simulink model "SpacecraftDisturbances"  (Simulink 8.5)
settings: Solver=ode4  StartTime=0.0  StopTime=20000  FixedStep=1  RelTol=1e-3
InitFcn:
  | % Bifocal Relay Mirror Spacecraft (prior to payload installation) Dynamics Simulation      TA Sands
  | clear all;close all;clc;warning off all;
  | 
  | % Simulation run parameters
  | Rate=34.3; DeltaT=1/Rate;
  | 
  | % Maneuver Parameters
  | roll=0; pitch=0; yaw=30; roll=roll*pi/180; pitch=pitch*pi/180; yaw=yaw*pi/180;
  | SlewTime=5; SACengage=0;
  | 
  | %Constants0
  | Re=6371.2e3;mu=398601.2e9; %earth radius and universal gravitation constant
  | 
  | %Spacecraft orbit
  | h=300e3; %orbit altitude in meters
  | R=Re+h; %orbit radius from center of earth
  | we=0.000072921158553; %earth's angular velocity rad/solar sec(Vallado)
  | wo=sqrt(mu/(Re+h)^3); %orbit angular velocity
  | incln=36.6001*pi/180; %Inclination assumed Monterey Latitude
  | epsilon=12*pi/180; alphao=0;
  | uo=0; nuo=0; %Start S/C beneath subsolar point
  | beta=60; gamma=1.5;
  | a=0.545491852; b=0.314939867; c=0.704226952; %Assumed spacecraft rectangular size
  | Area=[b*c a*c a*b]; %projected area~m^2 in body x,y,z directions
  | density=4.39e-14;
  | kpre=-9.9639/24/3600/180*pi*0; %nodal precession constant assumed zero here
  | wn=kpre*(Re/(Re+h))^3.5*cos(incln); %nodal precession (zero eccentricity)
  | V=wo*(Re+h);
  | rho=asin(Re/(h+Re)); %earth angular radius
  | Cd=2.5; psun=4.5E-6; %Drag coefficient and solar pressure constant~N/m^2
  | Kaero=-0.5*Cd*V^2; Psolar=2*psun; %constants for aero and solar torque calculation
  | dL=[0.002 0.002 0.008]; %predicted distance between cp and cg
  | Kme=2.3390e-005;
  | 
  | %Spacecraft Magnetic Properties (assumed)
  | mresid=[0 0 0.01]; %Spacecraft residual magnetic moment
  | M=mresid; %Magnetic unit dipole vector
  | K=7.943e15;
  | MBF=K/R^3;
  | 
  | %Spacecraft Inertia conditions
  | Ix=119.1259; Iy=150.6615; Iz=106.0288;
  | Ixy=-15.76781; Iyz=22.3164; Ixz=-6.5486;
  | %Ixy=0;Iyz=0;Ixz=0;
  | Imo=[Ix Ixy Ixz;
  | Ixy Iy Iyz;
  | Ixz Iyz Iz]; %Moment of inertia matrix
  | Iinv=inv(Imo); %Moment of inertia inverse goes in dynamics block
  | 
  | %Spacecraft initial Euler state angles and rates
  | phio=0;thetao=0;psio=0; %Initial Euler Angles
  | phidoto=0;thetadoto=0;psidoto=0; %Initial Euler Rates
  | 
  | %Calculation of initial quaternion (qo) and angular momentum (Ho)
  | s1=sin(phio/2);s2=sin(thetao/2);s3=sin(psio/2);c1=cos(phio/2);c2=cos(thetao/2);c3=cos(psio/2);
  | q1o=s1*c2*c3-c1*s2*s3;
  | q2o=c1*s2*c3+s1*c2*s3; %Wie pg. 321
  | q3o=c1*c2*s3-s1*s2*c3;
  | q4o=c1*c2*c3+s1*s2*s3;
  | S1=sin(phio);S2=sin(thetao);S3=sin(psio);C1=cos(phio);C2=cos(thetao);C3=cos(psio);
  | wxo=phidoto-psidoto*S2-wo*S3*C2;
  | wyo=thetadoto*C1+psidoto*C2*S1-wo*(C3*C1+S3*S2*S1);
  | wzo=psidoto*C2*C1-thetadoto*S1-wo*(S3*S2*C1-C3*S1);
  | qo=[q1o q2o q3o q4o];
  | Ho=Imo*[wxo wyo wzo]';
  | norm(Ho)*1000;
  | 
  | %Calculate eclipse time for comparison with EPS calculations
  | Te=100.87*2*V/2/pi;
  | 
  | 
  | 
StopFcn:
  | h2=figure;
  | plot(clock,Euler),title('Not Diagonal Inertia Matrix Euler Angles'),xlabel('time(sec)'),ylabel('Angles (degrees)'),grid
  | 
  | h3=figure;
  | plot(clock,Disturbances),title('Disturbances'),xlabel('time(sec)'),ylabel('torque'),grid
  | 
  | 
  | figure(3);
  | 
  | EulerX=Euler(:,1);EulerY=Euler(:,2);EulerZ=Euler(:,3);
  | subplot(4,1,1);plot(clock,EulerX,'linewidth',3); axis([0,20000,min(EulerX)-0.01,max(EulerX)+0.01]);grid;ylabel('\phi(deg)','fontsize',14);title('True Euler Angles','fontsize',14); set(gca,'XTickLabel',{' ',' ',' ',' ',' ',' ',' ',' ','15'}); set(gca,'fontsize',16);
  | subplot(4,1,2);plot(clock,EulerY,'linewidth',3); axis([0,20000,min(EulerY)-0.01,max(EulerY)+0.01]); grid;ylabel('\theta(deg)','fontsize',14); set(gca,'XTickLabel',{' ',' ',' ',' ',' ',' ',' ',' ','15'}); set(gca,'fontsize',16);
  | subplot(4,1,3);plot(clock,EulerZ,'linewidth',3);axis([0,20000,min(EulerZ)-0.01,max(EulerZ)+0.01]);grid; ylabel('\psi(deg)','fontsize',14); set(gca,'XTickLabel',{' ',' ',' ',' ',' ',' ',' ',' ','15'}); set(gca,'fontsize',16);
  | 
  | EX=ERROR(:,1); EY=ERROR(:,2); EZ=ERROR(:,3);
  | MeanXerror=mean(EX); Xmean=num2str(MeanXerror); xmean=['\mu_\phi=', Xmean];
  | STDx=std(EX);Xsigma=num2str(STDx);SigmaX=[' \sigma_x=' Xsigma]; xlegend=[xmean, SigmaX];
  | MeanYerror=mean(EY); Ymean=num2str(MeanYerror); ymean=['\mu_\theta=', Ymean];
  | STDy=std(EY); Ysigma=num2str(STDy);SigmaY=[' \sigma_y=' Ysigma]; ylegend=[ymean, SigmaY];
  | MeanZerror=mean(EZ); Zmean=num2str(MeanZerror); zmean=['\mu_\psi=', Zmean];
  | STDz=std(EZ);Zsigma=num2str(STDz);SigmaZ=[' \sigma_z=' Zsigma]; zlegend=[zmean, SigmaZ];
  | MeanError=[MeanXerror MeanYerror MeanZerror]; StdDev=[STDx STDy STDz];
  | 
  | 
  | subplot(4,1,1);plot(clock,EulerX,'linewidth',2); axis([0,20000,min(EulerX)-0.01,max(EulerX)+0.01]);grid;ylabel('\phi(deg)','fontsize',10);title('Standard Deviation Euler Angles','fontsize',14); set(gca,'XTickLabel',{' ',' ',' ',' ',' ',' ',' ',' ','10'}); set(gca,'fontsize',10);
  | subplot(4,1,2);plot(clock,EulerY,'linewidth',2); axis([0,20000,min(EulerY)-0.01,max(EulerY)+0.01]); grid;ylabel('\theta(deg)','fontsize',10); set(gca,'XTickLabel',{' ',' ',' ',' ',' ',' ',' ',' ','10'}); set(gca,'fontsize',10);
  | subplot(4,1,3);plot(clock,EulerZ,'linewidth',2);axis([0,20000,min(EulerZ)-0.01,max(EulerZ)+0.01]);grid; ylabel('\psi(deg)','fontsize',10); set(gca,'XTickLabel',{' ',' ',' ',' ',' ',' ',' ',' ','10'}); set(gca,'fontsize',10);
  | subplot(4,1,4);plot(clock,EulerX,'linewidth',2);axis([0,20000,min(EulerZ)-0.01,max(EulerZ)+0.01]);grid; ylabel('\psi(deg)','fontsize',10); set(gca,'XTickLabel',{' ',' ',' ',' ',' ',' ',' ',' ','10'}); set(gca,'fontsize',10);
  | 
  | 
  | figure(7);
  | 
  | EulerX=Euler(:,1);EulerY=Euler(:,2);EulerZ=Euler(:,3);
  | 
  | subplot(3,1,1);plot(clock,EulerX,'linewidth',1.5); axis([0,20000,min(EulerX)-10,max(EulerX)+10]);grid;ylabel('roll(deg)','fontsize',10);title('Euler Angles','fontsize',14); set(gca,'XTickLabel'); set(gca,'fontsize',10);
  | subplot(3,1,2);plot(clock,EulerY,'linewidth',1.5); axis([0,20000,min(EulerY)-10,max(EulerY)+10]); grid;ylabel('pitch(deg)','fontsize',10); set(gca,'XTickLabel'); set(gca,'fontsize',10);
  | subplot(3,1,3);plot(clock,EulerZ,'linewidth',1.5);axis([0,20000,min(EulerZ)-10,max(EulerZ)+10]);grid; ylabel('yaw(deg)','fontsize',10); set(gca,'XTickLabel'); set(gca,'fontsize',10);
  | 
  | figure(8);
  | 
  | DistX=Disturbances(:,1);DistY=Disturbances(:,2);DistZ=Disturbances(:,3);
  | 
  | subplot(3,1,1);plot(clock,DistX,'linewidth',1.5); axis([0,20000,min(DistX)-0.000001,max(DistX)+0.000001]);grid;ylabel('roll(deg)','fontsize',10);title('Disturbances','fontsize',14); set(gca,'XTickLabel'); set(gca,'fontsize',10);
  | subplot(3,1,2);plot(clock,DistY,'linewidth',1.5);axis([0,20000,min(DistY)-0.000001,max(DistY)+0.000001]);grid; ylabel('pitch(deg)','fontsize',10); set(gca,'XTickLabel'); set(gca,'fontsize',10);
  | subplot(3,1,3);plot(clock,DistZ,'linewidth',1.5);axis([0,20000,min(DistZ)-0.000001,max(DistZ)+0.000001]);grid; ylabel('yaw(deg)','fontsize',10); set(gca,'XTickLabel'); set(gca,'fontsize',10);
  | 
  | figure(9);
  | 
  | GravX=Gravity(:,1);GravY=Gravity(:,2);GravZ=Gravity(:,3);
  | 
  | subplot(3,1,1);plot(clock,GravX,'linewidth',1.5); axis([0,20000,min(GravX)-0.000001,max(GravX)+0.000001]);grid;ylabel('roll(deg)','fontsize',10);title('Gravity Gradient','fontsize',14); set(gca,'XTickLabel'); set(gca,'fontsize',10);
  | subplot(3,1,2);plot(clock,GravY,'linewidth',1.5);axis([0,20000,min(GravY)-0.000001,max(GravY)+0.000001]);grid; ylabel('pitch(deg)','fontsize',10); set(gca,'XTickLabel'); set(gca,'fontsize',10);
  | subplot(3,1,3);plot(clock,GravZ,'linewidth',1.5);axis([0,20000,min(GravZ)-0.000001,max(GravZ)+0.000001]);grid; ylabel('yaw(deg)','fontsize',10); set(gca,'XTickLabel'); set(gca,'fontsize',10);
  | 
  | figure(10);
  | 
  | MagX=Magnetic(:,1);MagY=Magnetic(:,2);MagZ=Magnetic(:,3);
  | 
  | subplot(3,1,1);plot(clock,MagX,'linewidth',1.5); axis([0,20000,min(MagX)-0.000000001,max(MagX)+0.000000001]);grid;ylabel('roll(deg)','fontsize',10);title('Magnetic Torque','fontsize',14); set(gca,'XTickLabel'); set(gca,'fontsize',10);
  | subplot(3,1,2);plot(clock,MagY,'linewidth',1.5);axis([0,20000,min(MagY)-0.000000001,max(MagY)+0.000000001]);grid; ylabel('pitch(deg)','fontsize',10); set(gca,'XTickLabel'); set(gca,'fontsize',10);
  | subplot(3,1,3);plot(clock,MagZ,'linewidth',1.5);axis([0,20000,min(MagZ)-0.000000001,max(MagZ)+0.000000001]);grid; ylabel('yaw(deg)','fontsize',10); set(gca,'XTickLabel'); set(gca,'fontsize',10);
  | 
  | figure(11);
  | 
  | ASX=AeroSolar(:,1);ASY=AeroSolar(:,2);ASZ=AeroSolar(:,3);
  | 
  | subplot(3,1,1);plot(clock,ASX,'linewidth',1.5); axis([0,20000,min(ASX)-0.000001,max(ASX)+0.000001]);grid;ylabel('roll(deg)','fontsize',10);title('AeroDynamic & Solar Disturbances','fontsize',14); set(gca,'XTickLabel'); set(gca,'fontsize',10);
  | subplot(3,1,2);plot(clock,ASY,'linewidth',1.5);axis([0,20000,min(ASY)-0.000001,max(ASY)+0.000001]);grid; ylabel('pitch(deg)','fontsize',10); set(gca,'XTickLabel'); set(gca,'fontsize',10);
  | subplot(3,1,3);plot(clock,ASZ,'linewidth',1.5);axis([0,20000,min(ASZ)-0.000001,max(ASZ)+0.000001]);grid; ylabel('yaw(deg)','fontsize',10); set(gca,'XTickLabel'); set(gca,'fontsize',10);
  | 
  | figure(11);
  | 
  | AX=Gravity(:,1);AY=Magnetic(:,1);AZ=AeroSolar(:,1);
  | 
  | subplot(3,1,1);plot(clock,AX,'linewidth',1.5); axis([0,20000,min(AX),max(AX)]);grid;ylabel('Gravity','fontsize',10);title('Disturbances on Roll','fontsize',14); set(gca,'XTickLabel'); set(gca,'fontsize',10);
  | subplot(3,1,2);plot(clock,AY,'linewidth',1.5);axis([0,20000,min(AY),max(AY)]);grid; ylabel('Magnetic','fontsize',10); set(gca,'XTickLabel'); set(gca,'fontsize',10);
  | subplot(3,1,3);plot(clock,AZ,'linewidth',1.5);axis([0,20000,min(AZ),max(AZ)]);grid; ylabel('Aerosolar','fontsize',10); set(gca,'XTickLabel'); set(gca,'fontsize',10);
  | 
  | figure(5);
  | 
  | DX=art(:,2);DY=art(:,3);DZ=art(:,4);
  | 
  | subplot(3,1,1);plot(clock,DX,'linewidth',1.5); axis([0,20000,min(DX)-0.000001,max(DX)+0.000001]);grid;ylabel('step','fontsize',10);title('Disturbances','fontsize',14); set(gca,'XTickLabel'); set(gca,'fontsize',10);
  | subplot(3,1,2);plot(clock,DY,'linewidth',1.5);axis([0,20000,min(DY)-0.000001,max(DY)+0.000001]);grid; ylabel('pulse','fontsize',10); set(gca,'XTickLabel'); set(gca,'fontsize',10);
  | subplot(3,1,3);plot(clock,DZ,'linewidth',1.5);axis([0,20000,min(DZ)-0.000001,max(DZ)+0.000001]);grid; ylabel('sine','fontsize',10); set(gca,'XTickLabel'); set(gca,'fontsize',10);
  | 
  | 
  | figure(14)
  | 
  | subplot(3,1,1) ;plot(clock,ERROR(:,1)*180/pi,'linewidth',3); set(gca,'fontsize',10);title('Euler Angles','fontsize',14); ylabel('\phi Degrees','fontsize',10);
  | legend(['angle','  \mu=',num2str(mean(ERROR(:,1))),'  \sigma=',num2str(std(ERROR(:,1)))],'Location','Best')
  | legend('boxoff')
  | grid on
  | set(gca,'XTickLabel',{})
  | 
  | subplot(3,1,2) ;plot(clock,ERROR(:,2)*180/pi,'linewidth',3) ;set(gca,'fontsize',10);ylabel('\theta Degrees','fontsize',10) ;
  | legend(['angle','  \mu=',num2str(mean(ERROR(:,2))),'  \sigma=',num2str(std(ERROR(:,2)))],'Location','Best') ;
  | legend('boxoff')
  | grid on
  | set(gca,'XTickLabel',{})
  | 
  | subplot(3,1,3) ;plot(clock,ERROR(:,3)*180/pi,'linewidth',3) ;set(gca,'fontsize',10);ylabel('\psi Degrees','fontsize',10) ;xlabel('Time (s)','fontsize',10) ;
  | legend(['angle','  \mu=',num2str(mean(ERROR(:,3))),'  \sigma=',num2str(std(ERROR(:,3)))],'Location','Best')
  | legend('boxoff')
  | grid on
libraries: aerospace x4, vrlib x1, simulink x1
settings Model: Creator=grompone  LastModifiedBy=Acer
settings OptimizationCC: InitFltsAndDblsToZero=on
settings DebuggingCC: SaveWithParameterizedLinksMsg=none  SolverPrmCheckMsg=warning  FcnCallInpInsideContextMsg=UseLocalSettings  StrictBusMsg=Warning
settings SFSimCC: SimParseCustomCode=off
settings GRTTargetCC: TargetFcnLib=ansi_tfl_tmw.mat

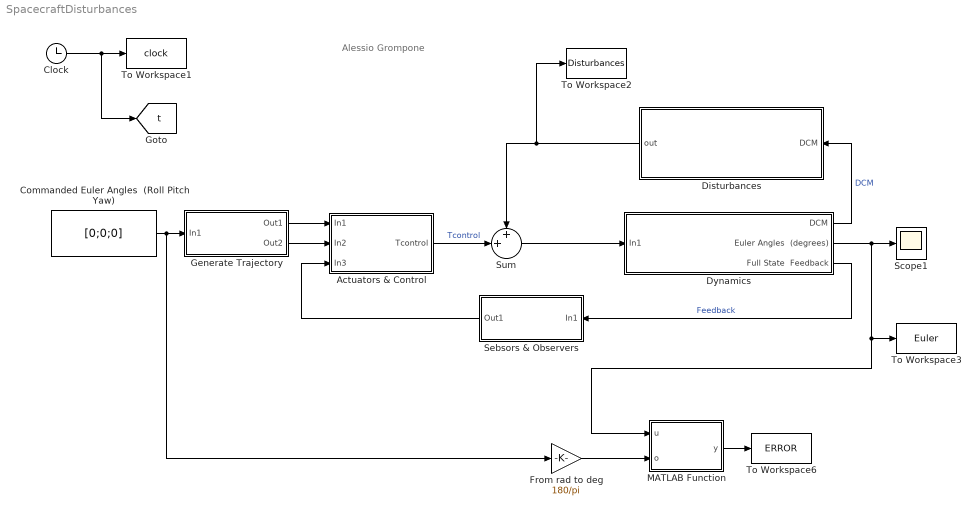
== system SpacecraftDisturbances ==
  note: Alessio Grompone
  Actuators & Control : Subsystem
  Clock : Clock
  Commanded Euler Angles  (Roll Pitch Yaw) : Constant  Value=[0;0;0]
  Disturbances : Subsystem
  Dynamics : Subsystem
  From rad to deg : Gain  Gain=180/pi
  Generate Trajectory : Subsystem
  MATLAB Function : MATLAB Function  TreatAsAtomicUnit=on
  Scope1 : Scope
      settings: SaveName=ScopeData2
  Sebsors & Observers : Subsystem
  Sum : Sum  Inputs=++|
  To Workspace1 : ToWorkspace  VariableName=clock  SampleTime=-1
  To Workspace2 : ToWorkspace  VariableName=Disturbances  SampleTime=-1
  To Workspace3 : ToWorkspace  VariableName=Euler  SampleTime=-1
  To Workspace6 : ToWorkspace  VariableName=ERROR  SampleTime=-1
  tag scope: t=global
  wires:
  Clock/1 -> To Workspace1/1, [t]
  Sum/1 -> Dynamics/1(In1)
  Commanded Euler Angles  (Roll Pitch Yaw)/1 -> Generate Trajectory/1(In1), From rad to deg/1
  Generate Trajectory/1(Out1) -> Actuators & Control/1(In1)
  Generate Trajectory/2(Out2) -> Actuators & Control/2(In2)
  Sebsors & Observers/1(Out1) -> Actuators & Control/3(In3)
  Dynamics/2(Euler Angles  (degrees)) -> Scope1/1, To Workspace3/1, MATLAB Function/1(u)
  Dynamics/1(DCM) -> Disturbances/1(DCM)  "DCM"
  Dynamics/3(Full State  Feedback) -> Sebsors & Observers/1(In1)  "Feedback"
  Disturbances/1(out) -> Sum/1, To Workspace2/1
  Actuators & Control/1(Tcontrol) -> Sum/2  "Tcontrol"
  MATLAB Function/1(y) -> To Workspace6/1
  From rad to deg/1 -> MATLAB Function/2(o)

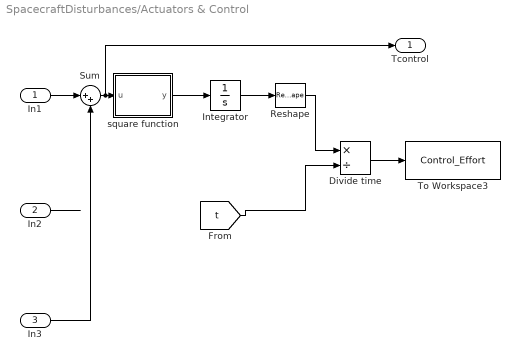
== system SpacecraftDisturbances/Actuators & Control ==
  In1 : Inport
  In2 : Inport  Port=2
  In3 : Inport  Port=3
  Divide time : Product  Inputs=*/
  Integrator : Integrator
  Reshape : Reshape
  Sum : Sum  Inputs=|++
  To Workspace3 : ToWorkspace  VariableName=Control_Effort  SampleTime=-1
  square function : MATLAB Function  TreatAsAtomicUnit=on
  Tcontrol : Outport
  wires:
  [t] -> Divide time/2
  square function/1(y) -> Integrator/1
  Integrator/1 -> Reshape/1
  Divide time/1 -> To Workspace3/1
  Reshape/1 -> Divide time/1
  In2/1 -> ?
  In1/1 -> Sum/1
  In3/1 -> Sum/2
  Sum/1 -> square function/1(u), Tcontrol/1

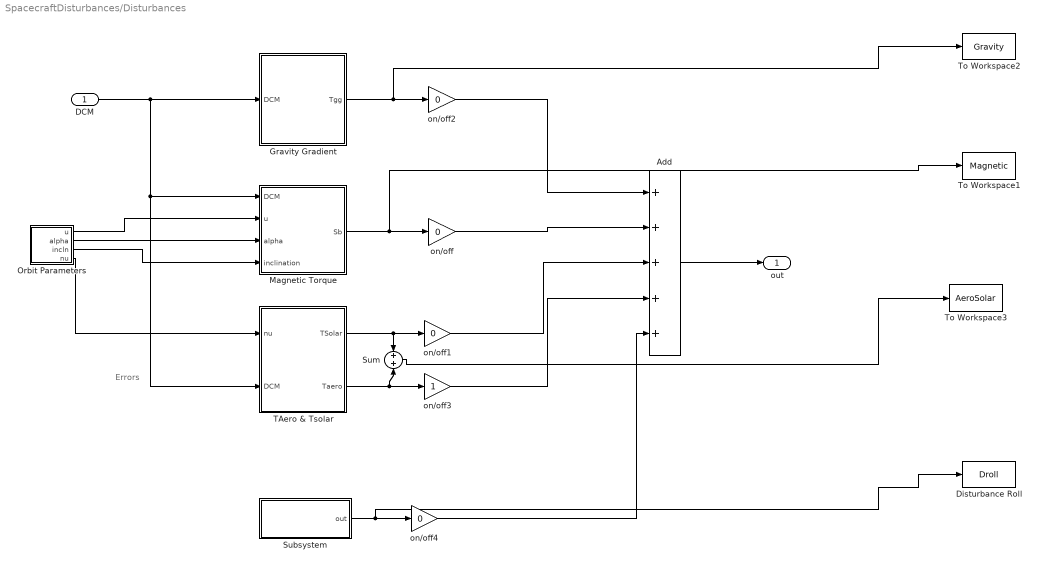
== system SpacecraftDisturbances/Disturbances ==
  note: Errors
  DCM : Inport
  Add : Sum  Inputs=+++++
  Disturbance Roll : ToWorkspace  VariableName=Droll  SampleTime=-1
  Gravity Gradient : Subsystem
  Magnetic Torque : Subsystem
  Orbit Parameters : Subsystem
  Subsystem : Subsystem
  Sum : Sum  Inputs=+|+
  TAero & Tsolar : Subsystem
  To Workspace1 : ToWorkspace  VariableName=Magnetic  SampleTime=-1
  To Workspace2 : ToWorkspace  VariableName=Gravity  SampleTime=-1
  To Workspace3 : ToWorkspace  VariableName=AeroSolar  SampleTime=-1
  on/off{,1..2,4} (4 alike) : Gain  Gain=0
  on/off3 : Gain
  out : Outport
  wires:
  DCM/1 -> Magnetic Torque/1(DCM), TAero & Tsolar/2(DCM), Gravity Gradient/1(DCM)
  TAero & Tsolar/1(TSolar) -> on/off1/1, Sum/1
  Magnetic Torque/1(Sb) -> on/off/1, To Workspace1/1
  Orbit Parameters/1(u) -> Magnetic Torque/2(u)
  Orbit Parameters/2(alpha) -> Magnetic Torque/3(alpha)
  Orbit Parameters/3(incln) -> Magnetic Torque/4(inclination)
  Orbit Parameters/4(nu) -> TAero & Tsolar/1(nu)
  Gravity Gradient/1(Tgg) -> on/off2/1, To Workspace2/1
  Add/1 -> out/1
  on/off2/1 -> Add/1
  on/off/1 -> Add/2
  TAero & Tsolar/2(Taero) -> on/off3/1, Sum/2
  on/off1/1 -> Add/3
  on/off3/1 -> Add/4
  Subsystem/1(out) -> on/off4/1, Disturbance Roll/1
  on/off4/1 -> Add/5
  Sum/1 -> To Workspace3/1

== system SpacecraftDisturbances/Dynamics ==
  In1 : Inport
  Dynamics : Subsystem
  Kinematics : Subsystem
  Mux : Mux  Inputs=2
  DCM : Outport
  Euler Angles  (degrees) : Outport  Port=2
  Full State  Feedback : Outport  Port=3
  wires:
  Dynamics/1(w_nb) -> Kinematics/1(w_nb), Mux/2
  Kinematics/1(DCM) -> DCM/1
  In1/1 -> Dynamics/1(taug)
  Kinematics/2(Euler Angles  (degrees)) -> Euler Angles  (degrees)/1
  Mux/1 -> Full State  Feedback/1
  Kinematics/3(Euler Angles) -> Mux/1

== system SpacecraftDisturbances/Generate Trajectory ==
  In1 : Inport
  Out1 : Outport
  Out2 : Outport  Port=2
  wires:
  In1/1 -> Out1/1

== system SpacecraftDisturbances/Sebsors & Observers ==
  In1 : Inport
  Demux : Demux  Outputs=6
  Mux : Mux  Inputs=3
  Out1 : Outport
  wires:
  Mux/1 -> Out1/1
  Demux/1 -> Mux/1
  Demux/2 -> Mux/2
  Demux/3 -> Mux/3

== system SpacecraftDisturbances/Disturbances/Gravity Gradient ==
  DCM : Inport
  3*mu/Ro^3 : Gain  Gain=3*mu/(h+Re)^3  Multiplication=Matrix(K*u)  SaturateOnIntegerOverflow=on  OutDataTypeStr=Inherit: Same as input  ParamDataTypeStr=Inherit: Same as input
  3x3 cross product : aerospace/Axes Transformations/3x3 cross product
  Ib : Gain  Gain=Imo  Multiplication=Matrix(K*u)  SaturateOnIntegerOverflow=on  OutDataTypeStr=Inherit: Same as input  ParamDataTypeStr=Inherit: Same as input
  Select ci3 : Subsystem
  Tgg : Outport
  wires:
  Ib/1 -> 3x3 cross product/2
  3*mu/Ro^3/1 -> Tgg/1
  3x3 cross product/1 -> 3*mu/Ro^3/1
  Select ci3/1(U(E)) -> 3x3 cross product/1, Ib/1
  DCM/1 -> Select ci3/1(U)

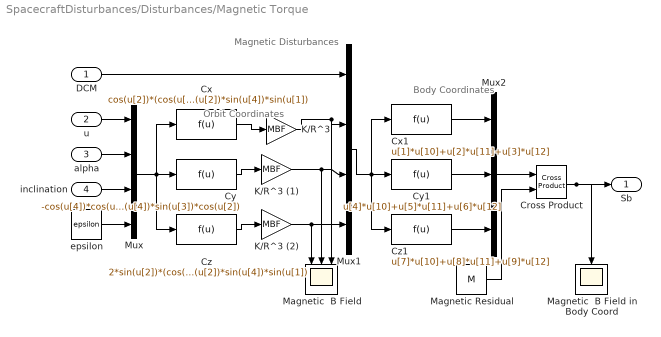
== system SpacecraftDisturbances/Disturbances/Magnetic Torque ==
  note: Magnetic Disturbances
  note: Orbit Coordinates
  note: Body Coordinates
  DCM : Inport
  u : Inport  Port=2
  alpha : Inport  Port=3
  inclination : Inport  Port=4
  Cross Product : vrlib/Utilities/Cross Product
  Cx : Fcn  Expr=cos(u[2])*(cos(u[4])*sin(u[3])-sin(u[4])*cos(u[3])*cos(u[1]))-sin(u[2])*sin(u[4])*sin(u[1])
  Cx1 : Fcn  Expr=u[1]*u[10]+u[2]*u[11]+u[3]*u[12]
  Cy : Fcn  Expr=-cos(u[4])*cos(u[3])-sin(u[4])*sin(u[3])*cos(u[2])
  Cy1 : Fcn  Expr=u[4]*u[10]+u[5]*u[11]+u[6]*u[12]
  Cz : Fcn  Expr=2*sin(u[2])*(cos(u[4])*sin(u[3])-sin(u[4])*cos(u[3])*cos(u[1]))+2*cos(u[2])*sin(u[4])*sin(u[1])
  Cz1 : Fcn  Expr=u[7]*u[10]+u[8]*u[11]+u[9]*u[12]
  K/R^3 : Gain  Gain=MBF
  K/R^3 (1) : Gain  Gain=MBF
  K/R^3 (2) : Gain  Gain=MBF
  Magnetic Residual : Constant  Value=M
  Magnetic  B Field : Scope  NumInputPorts=3
      settings: YMin=-5~-5~-5  YMax=5~5~5  SaveName=ScopeData3
  Magnetic  B Field in Body Coord : Scope
      settings: SaveName=ScopeData4
  Mux : Mux
  Mux1 : Mux
  Mux2 : Mux  Inputs=3
  epsilon : Constant  Value=epsilon
  Sb : Outport
  wires:
  u/1 -> Mux/1
  inclination/1 -> Mux/3
  alpha/1 -> Mux/2
  Cx/1 -> K/R^3/1
  Cy/1 -> K/R^3 (1)/1
  Cz/1 -> K/R^3 (2)/1
  DCM/1 -> Mux1/1
  Mux/1 -> Cy/1, Cz/1, Cx/1
  K/R^3/1 -> Mux1/2, Magnetic  B Field/3
  K/R^3 (1)/1 -> Mux1/3, Magnetic  B Field/2
  K/R^3 (2)/1 -> Mux1/4, Magnetic  B Field/1
  epsilon/1 -> Mux/4
  Mux1/1 -> Cy1/1, Cz1/1, Cx1/1
  Cx1/1 -> Mux2/1
  Cy1/1 -> Mux2/2
  Cz1/1 -> Mux2/3
  Magnetic Residual/1 -> Cross Product/2
  Mux2/1 -> Cross Product/1
  Cross Product/1 -> Sb/1, Magnetic  B Field in Body Coord/1

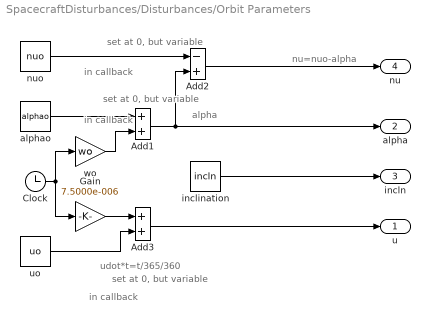
== system SpacecraftDisturbances/Disturbances/Orbit Parameters ==
  note: nu=nuo-alpha
  note: alpha
  note: udot*t=t/365/360
  note: set at 0, but variable
  note: in callback
  note: set at 0, but variable
  note: in callback
  note: set at 0, but variable
  note: in callback
  Add1 : Sum
  Add2 : Sum  Inputs=-+
  Add3 : Sum
  Clock : Clock
  Gain : Gain  Gain=7.5000e-006
  alphao : Constant  Value=alphao
  inclination : Constant  Value=incln
  nuo : Constant  Value=nuo
  uo : Constant  Value=uo
  wo : Gain  Gain=wo
  u : Outport
  alpha : Outport  Port=2
  incln : Outport  Port=3
  nu : Outport  Port=4
  wires:
  nuo/1 -> Add2/1
  Add2/1 -> nu/1
  alphao/1 -> Add1/1
  Clock/1 -> wo/1, Gain/1
  wo/1 -> Add1/2
  Add1/1 -> alpha/1, Add2/2
  uo/1 -> Add3/2
  Gain/1 -> Add3/1
  inclination/1 -> incln/1
  Add3/1 -> u/1

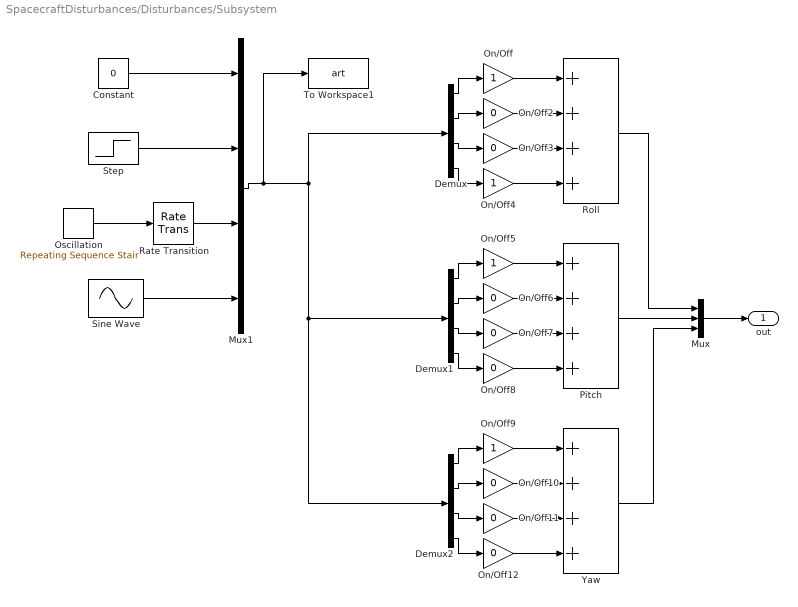
== system SpacecraftDisturbances/Disturbances/Subsystem ==
  Constant : Constant  Value=0
  Demux : Demux
  Demux1 : Demux
  Demux2 : Demux
  Mux : Mux  Inputs=3
  Mux1 : Mux
  On/Off{,4..5,9} (4 alike) : Gain  SaturateOnIntegerOverflow=on  OutDataTypeStr=Inherit: Same as input  ParamDataTypeStr=Inherit: Same as input
  On/Off{2..3,6..8,10..12} (8 alike) : Gain  Gain=0  SaturateOnIntegerOverflow=on  OutDataTypeStr=Inherit: Same as input  ParamDataTypeStr=Inherit: Same as input
  Oscillation : simulink/Sources/Repeating Sequence Stair  OutValues=[ 0.01 -0.01 -0.01 0.01]  tsamp=1000  OutMin=[]  OutMax=[]  OutDataTypeStr=double  OutputDataTypeScalingMode=double  OutDataType=fixdt(0,8)  ConRadixGroup=Best Precision: Vector-wise  OutScaling=2^-12
  Pitch : Sum  Inputs=++++
  Rate Transition : RateTransition
  Roll : Sum  Inputs=++++
  Sine Wave : Sin  Amplitude=.1  Frequency=1000  SampleTime=0  VectorParams1D=off
  Step : Step  Time=4000  After=0.1  SampleTime=0
  To Workspace1 : ToWorkspace  VariableName=art  SampleTime=-1
  Yaw : Sum  Inputs=++++
  out : Outport
  wires:
  On/Off/1 -> Roll/1
  On/Off2/1 -> Roll/2
  On/Off3/1 -> Roll/3
  On/Off4/1 -> Roll/4
  On/Off5/1 -> Pitch/1
  On/Off6/1 -> Pitch/2
  On/Off7/1 -> Pitch/3
  On/Off8/1 -> Pitch/4
  On/Off9/1 -> Yaw/1
  On/Off10/1 -> Yaw/2
  On/Off11/1 -> Yaw/3
  On/Off12/1 -> Yaw/4
  Roll/1 -> Mux/1
  Pitch/1 -> Mux/2
  Yaw/1 -> Mux/3
  Demux/1 -> On/Off/1
  Demux/2 -> On/Off2/1
  Demux/3 -> On/Off3/1
  Demux/4 -> On/Off4/1
  Demux1/1 -> On/Off5/1
  Demux1/2 -> On/Off6/1
  Demux1/3 -> On/Off7/1
  Demux1/4 -> On/Off8/1
  Demux2/1 -> On/Off9/1
  Demux2/2 -> On/Off10/1
  Demux2/3 -> On/Off11/1
  Demux2/4 -> On/Off12/1
  Constant/1 -> Mux1/1
  Step/1 -> Mux1/2
  Mux/1 -> out/1
  Mux1/1 -> Demux/1, Demux1/1, Demux2/1, To Workspace1/1
  Sine Wave/1 -> Mux1/4
  Rate Transition/1 -> Mux1/3
  Oscillation/1 -> Rate Transition/1

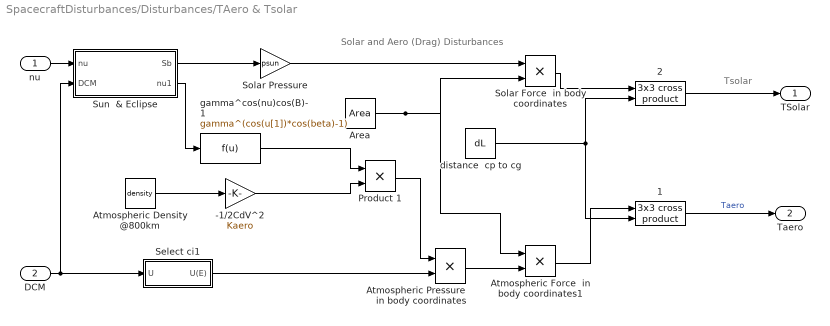
== system SpacecraftDisturbances/Disturbances/TAero & Tsolar ==
  note: Tsolar
  note: Solar and Aero (Drag) Disturbances
  nu : Inport
  DCM : Inport  Port=2
  -1/2CdV^2 : Gain  Gain=Kaero
  1 : aerospace/Axes Transformations/3x3 cross product
  2 : aerospace/Axes Transformations/3x3 cross product
  Area : Constant  Value=Area
  Atmospheric Density @800km : Constant  Value=density
  Atmospheric Force  in body coordinates1 : Product  RndMeth=Zero
  Atmospheric Pressure in body coordinates : Product  RndMeth=Zero
  Product 1 : Product  RndMeth=Zero
  Select ci1 : Subsystem
  Solar Force  in body coordinates : Product  RndMeth=Zero
  Solar Pressure : Gain  Gain=psun
  Sun  & Eclipse : Subsystem
  distance  cp to cg : Constant  Value=dL
  gamma^cos(nu)cos(B)-1 : Fcn  Expr=gamma^(cos(u[1])*cos(beta)-1)
  TSolar : Outport
  Taero : Outport  Port=2
  wires:
  DCM/1 -> Select ci1/1(U), Sun  & Eclipse/2(DCM)
  nu/1 -> Sun  & Eclipse/1(nu)
  Sun  & Eclipse/1(Sb) -> Solar Pressure/1
  Sun  & Eclipse/2(nu1) -> gamma^cos(nu)cos(B)-1/1
  Solar Pressure/1 -> Solar Force  in body coordinates/1
  gamma^cos(nu)cos(B)-1/1 -> Product 1/1
  Atmospheric Pressure in body coordinates/1 -> Atmospheric Force  in body coordinates1/2
  Atmospheric Density @800km/1 -> -1/2CdV^2/1
  -1/2CdV^2/1 -> Product 1/2
  Area/1 -> Solar Force  in body coordinates/2, Atmospheric Force  in body coordinates1/1
  Select ci1/1(U(E)) -> Atmospheric Pressure in body coordinates/2
  Product 1/1 -> Atmospheric Pressure in body coordinates/1
  Solar Force  in body coordinates/1 -> 2/1
  distance  cp to cg/1 -> 2/2, 1/2
  2/1 -> TSolar/1
  1/1 -> Taero/1  "Taero"
  Atmospheric Force  in body coordinates1/1 -> 1/1

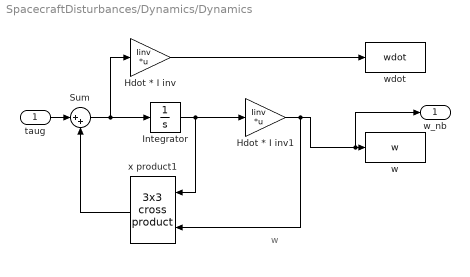
== system SpacecraftDisturbances/Dynamics/Dynamics ==
  note: w
  taug : Inport
  "  Hdot * I inv" : Gain  Gain=Iinv  Multiplication=Matrix(K*u)  SaturateOnIntegerOverflow=on  OutDataTypeStr=Inherit: Same as input  ParamDataTypeStr=Inherit: Same as input
  "  Hdot * I inv1" : Gain  Gain=Iinv  Multiplication=Matrix(K*u)  SaturateOnIntegerOverflow=on  OutDataTypeStr=Inherit: Same as input  ParamDataTypeStr=Inherit: Same as input
  Integrator : Integrator
  Sum : Sum  Inputs=|++
  w : ToWorkspace  VariableName=w  SampleTime=-1
  wdot : ToWorkspace  VariableName=wdot  SampleTime=-1
  x product1 : aerospace/Axes Transformations/3x3 cross product
  w_nb : Outport
  wires:
  Integrator/1 -> x product1/1, "  Hdot * I inv1"/1
  taug/1 -> Sum/1
  x product1/1 -> Sum/2
  Sum/1 -> "  Hdot * I inv"/1, Integrator/1
  "  Hdot * I inv"/1 -> wdot/1
  "  Hdot * I inv1"/1 -> x product1/2, w/1, w_nb/1

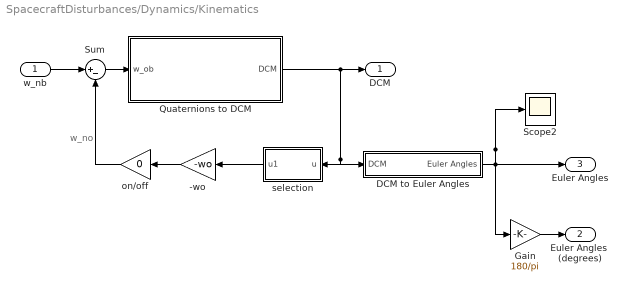
== system SpacecraftDisturbances/Dynamics/Kinematics ==
  note: w_no
  w_nb : Inport
  -wo : Gain  Gain=-wo
  DCM to Euler Angles : Subsystem
  Gain : Gain  Gain=180/pi
  Quaternions to DCM : Subsystem
  Scope2 : Scope
      settings: YMin=-60  YMax=60  SaveName=ScopeData3
  Sum : Sum  Inputs=|+-
  on/off : Gain  Gain=0
  "selection " : MATLAB Function  TreatAsAtomicUnit=on
  DCM : Outport
  Euler Angles  (degrees) : Outport  Port=2
  Euler Angles : Outport  Port=3
  wires:
  w_nb/1 -> Sum/1
  Quaternions to DCM/1(DCM) -> DCM/1, "selection "/1(u), DCM to Euler Angles/1(DCM)
  Sum/1 -> Quaternions to DCM/1(w_ob)
  on/off/1 -> Sum/2
  "selection "/1(u1) -> -wo/1
  -wo/1 -> on/off/1
  Gain/1 -> Euler Angles  (degrees)/1
  DCM to Euler Angles/1(Euler Angles) -> Scope2/1, Euler Angles/1, Gain/1

== system SpacecraftDisturbances/Disturbances/Gravity Gradient/Select ci3 ==
  U : Inport
  C13 : Fcn  Expr=u[3]
  C23 : Fcn  Expr=u[6]
  C33 : Fcn  Expr=u[9]
  Mux2 : Mux  Inputs=3
  U(E) : Outport
  wires:
  Mux2/1 -> U(E)/1
  U/1 -> C33/1, C13/1, C23/1
  C33/1 -> Mux2/3
  C23/1 -> Mux2/2
  C13/1 -> Mux2/1

== system SpacecraftDisturbances/Disturbances/TAero & Tsolar/Select ci1 ==
  U : Inport
  C13 : Fcn  Expr=u[1]
  C23 : Fcn  Expr=u[4]
  C33 : Fcn  Expr=u[7]
  Mux : Mux  Inputs=3
  U(E) : Outport
  wires:
  C23/1 -> Mux/2
  C13/1 -> Mux/1
  C33/1 -> Mux/3
  Mux/1 -> U(E)/1
  U/1 -> C13/1, C23/1, C33/1

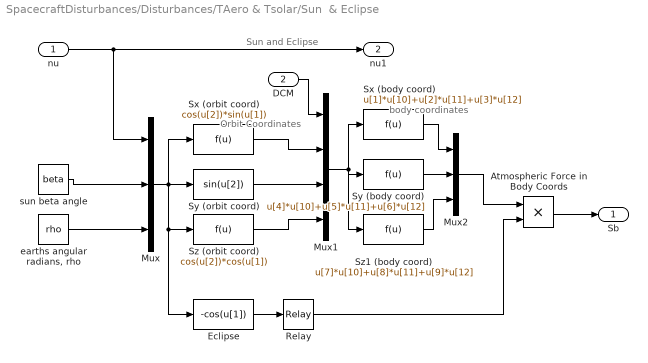
== system SpacecraftDisturbances/Disturbances/TAero & Tsolar/Sun  & Eclipse ==
  note: Sun and Eclipse
  note: Orbit Coordinates
  note: body coordinates
  nu : Inport
  DCM : Inport  Port=2
  Atmospheric Force in Body Coords : Product  RndMeth=Zero
  Eclipse : Fcn  Expr=-cos(u[1])
  Mux : Mux  Inputs=3
  Mux1 : Mux
  Mux2 : Mux  Inputs=3
  Relay : Relay  OnSwitchValue=cos(rho)/cos(beta)  OffSwitchValue=cos(rho)/cos(beta)-0.001  OnOutputValue=0  OffOutputValue=1
  Sx (body coord) : Fcn  Expr=u[1]*u[10]+u[2]*u[11]+u[3]*u[12]
  Sx (orbit coord) : Fcn  Expr=cos(u[2])*sin(u[1])
  Sy (body coord) : Fcn  Expr=u[4]*u[10]+u[5]*u[11]+u[6]*u[12]
  "Sy (orbit coord) " : Fcn  Expr=sin(u[2])
  Sz (orbit coord) : Fcn  Expr=cos(u[2])*cos(u[1])
  Sz1 (body coord) : Fcn  Expr=u[7]*u[10]+u[8]*u[11]+u[9]*u[12]
  "earths angular radians, rho" : Constant  Value=rho
  sun beta angle : Constant  Value=beta
  Sb : Outport
  nu1 : Outport  Port=2
  wires:
  Mux1/1 -> Sx (body coord)/1, Sy (body coord)/1, Sz1 (body coord)/1
  DCM/1 -> Mux1/1
  nu/1 -> nu1/1, Mux/1
  "earths angular radians, rho"/1 -> Mux/3
  sun beta angle/1 -> Mux/2
  Mux/1 -> "Sy (orbit coord) "/1, Sx (orbit coord)/1, Sz (orbit coord)/1, Eclipse/1
  Sx (orbit coord)/1 -> Mux1/2
  "Sy (orbit coord) "/1 -> Mux1/3
  Sz (orbit coord)/1 -> Mux1/4
  Atmospheric Force in Body Coords/1 -> Sb/1
  Sx (body coord)/1 -> Mux2/1
  Sy (body coord)/1 -> Mux2/2
  Sz1 (body coord)/1 -> Mux2/3
  Mux2/1 -> Atmospheric Force in Body Coords/1
  Eclipse/1 -> Relay/1
  Relay/1 -> Atmospheric Force in Body Coords/2

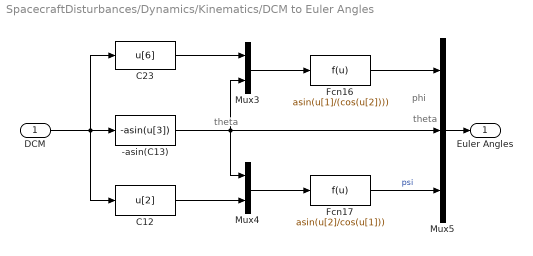
== system SpacecraftDisturbances/Dynamics/Kinematics/DCM to Euler Angles ==
  note: phi
  note: theta
  note: theta
  DCM : Inport
  -asin(C13) : Fcn  Expr=-asin(u[3])
  C12 : Fcn  Expr=u[2]
  C23 : Fcn  Expr=u[6]
      mask Display: disp('u[6]')
  Fcn16 : Fcn  Expr=asin(u[1]/(cos(u[2])))
  Fcn17 : Fcn  Expr=asin(u[2]/cos(u[1]))
  Mux3 : Mux  Inputs=2
  Mux4 : Mux  Inputs=2
  Mux5 : Mux  Inputs=3
  Euler Angles : Outport
  wires:
  Fcn16/1 -> Mux5/1
  Fcn17/1 -> Mux5/3  "psi"
  Mux5/1 -> Euler Angles/1
  C12/1 -> Mux4/2
  Mux4/1 -> Fcn17/1
  -asin(C13)/1 -> Mux5/2, Mux4/1, Mux3/2
  Mux3/1 -> Fcn16/1
  C23/1 -> Mux3/1
  DCM/1 -> -asin(C13)/1, C23/1, C12/1

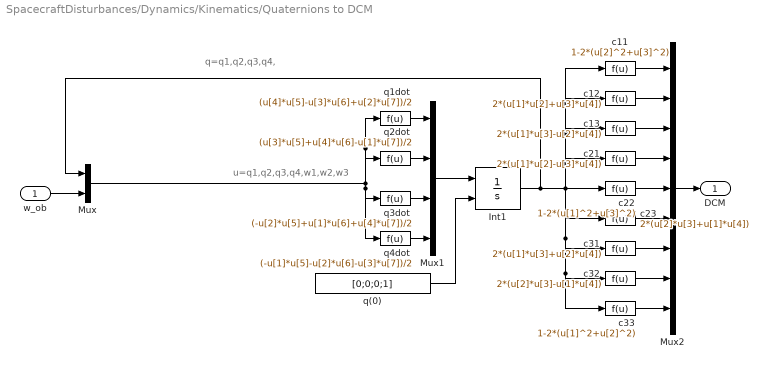
== system SpacecraftDisturbances/Dynamics/Kinematics/Quaternions to DCM ==
  note: q=q1,q2,q3,q4,
  note: u=q1,q2,q3,q4,w1,w2,w3
  w_ob : Inport
  Int1 : Integrator  InitialConditionSource=external  InitialCondition=[0 0 -0.1]'
  Mux : Mux  Inputs=2
  Mux1 : Mux
  Mux2 : Mux  Inputs=9
  c11 : Fcn  Expr=1-2*(u[2]^2+u[3]^2)
  c12 : Fcn  Expr=2*(u[1]*u[2]+u[3]*u[4])
  c13 : Fcn  Expr=2*(u[1]*u[3]-u[2]*u[4])
  c21 : Fcn  Expr=2*(u[1]*u[2]-u[3]*u[4])
  c22 : Fcn  Expr=1-2*(u[1]^2+u[3]^2)
  c23 : Fcn  Expr=2*(u[2]*u[3]+u[1]*u[4])
  c31 : Fcn  Expr=2*(u[1]*u[3]+u[2]*u[4])
  c32 : Fcn  Expr=2*(u[2]*u[3]-u[1]*u[4])
  c33 : Fcn  Expr=1-2*(u[1]^2+u[2]^2)
  q(0) : Constant  Value=[0;0;0;1]
  q1dot : Fcn  Expr=(u[4]*u[5]-u[3]*u[6]+u[2]*u[7])/2
  q2dot : Fcn  Expr=(u[3]*u[5]+u[4]*u[6]-u[1]*u[7])/2
  q3dot : Fcn  Expr=(-u[2]*u[5]+u[1]*u[6]+u[4]*u[7])/2
  q4dot : Fcn  Expr=(-u[1]*u[5]-u[2]*u[6]-u[3]*u[7])/2
  DCM : Outport
  wires:
  Mux/1 -> q4dot/1, q3dot/1, q1dot/1, q2dot/1
  q1dot/1 -> Mux1/1
  q2dot/1 -> Mux1/2
  q3dot/1 -> Mux1/3
  q4dot/1 -> Mux1/4
  Int1/1 -> Mux/1, c22/1, c21/1, c13/1, c12/1, c11/1, c23/1, c31/1, c32/1, c33/1
  Mux1/1 -> Int1/1
  q(0)/1 -> Int1/2
  c11/1 -> Mux2/1
  c12/1 -> Mux2/2
  c13/1 -> Mux2/3
  c21/1 -> Mux2/4
  c22/1 -> Mux2/5
  c23/1 -> Mux2/6
  c31/1 -> Mux2/7
  c32/1 -> Mux2/8
  c33/1 -> Mux2/9
  w_ob/1 -> Mux/2
  Mux2/1 -> DCM/1

== matlab function MATLAB Function ==
  data: u input double; y output double; o input double
function y = fcn(u,o)
%#codegen

y = u-o;

== matlab function Dynamics/Kinematics/selection  ==
  data: u input double; u1 output double
function u1  = Select(u)
% This block supports an embeddable subset of the MATLAB language.
% See the help menu for details. 

u11=u(2);

u22=u(5);

u33=u(8);

u1=[u11;u22;u33];

== matlab function Actuators & Control/square function ==
  data: u input double; y output double
function y = fcn(u)
%#codegen

y = u.^2;
